simulink model "plan_nika"  (R2021b)
settings: Solver=VariableStepAuto  StartTime=0.0  StopTime=100  RelTol=1e-3
values from neighbouring files (symbols this model uses):
  cren = 0    [sis_init.m]
  g = 9.8    [sis_init.m]
  speed_tgt = 100    [sis_init.m]
  speed_tgt_2 = 130    [sis_init.m]
  v0 = 20    [sis_init.m]
undefined symbols (not defined in the file or in its folder): h0, roll
settings Model: Creator=Acer  LastModifiedBy=Acer

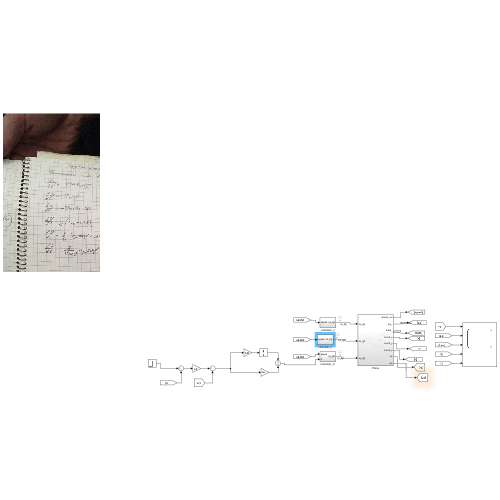
[thumbnail: Simulink's stored preview of the top-level diagram]
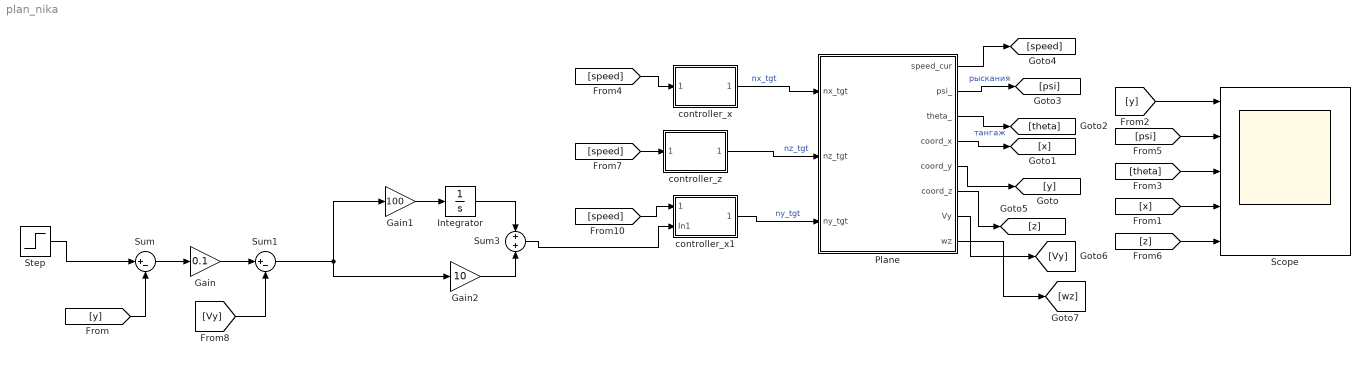
== system plan_nika ==
  Gain : Gain  Gain=0.1
  Gain1 : Gain  Gain=100
  Gain2 : Gain  Gain=10
  Integrator : Integrator
  Plane : Subsystem
  Scope : Scope  NumInputPorts=5
  Step : Step  Time=10  Before=h0  After=1500  SampleTime=0
  Sum : Sum  Inputs=|+-
  Sum1 : Sum  Inputs=|+-
  Sum3 : Sum  Inputs=+|+
  controller_x : Subsystem
  controller_x1 : Subsystem
  controller_z : Subsystem
  wires:
  controller_x/1(nx_tgt) -> Plane/1(nx_tgt)  "nx_tgt"
  Plane/5(coord_y) -> [y]
  Plane/2(psi_) -> [psi]  "рыскания"
  Plane/3(theta_) -> [theta]  "тангаж"
  Plane/4(coord_x) -> [x]
  Plane/1(speed_cur) -> [speed]
  [x] -> Scope/4
  [theta] -> Scope/3
  [speed] -> controller_x/1(speed)
  [psi] -> Scope/2
  Plane/6(coord_z) -> [z]
  [z] -> Scope/5
  [speed] -> controller_z/1(speed)
  controller_z/1(nz_tgt) -> Plane/2(nz_tgt)  "nz_tgt"
  [y] -> Scope/1
  controller_x1/1(ny_tgt) -> Plane/3(ny_tgt)  "ny_tgt"
  Step/1 -> Sum/1
  [y] -> Sum/2
  Sum/1 -> Gain/1
  Gain/1 -> Sum1/1
  Plane/7(Vy) -> [Vy]
  [Vy] -> Sum1/2
  Plane/8(wz) -> [wz]
  Integrator/1 -> Sum3/1
  Gain2/1 -> Sum3/2
  Gain1/1 -> Integrator/1
  Sum1/1 -> Gain1/1, Gain2/1
  Sum3/1 -> controller_x1/2(In1)
  [speed] -> controller_x1/1(speed)

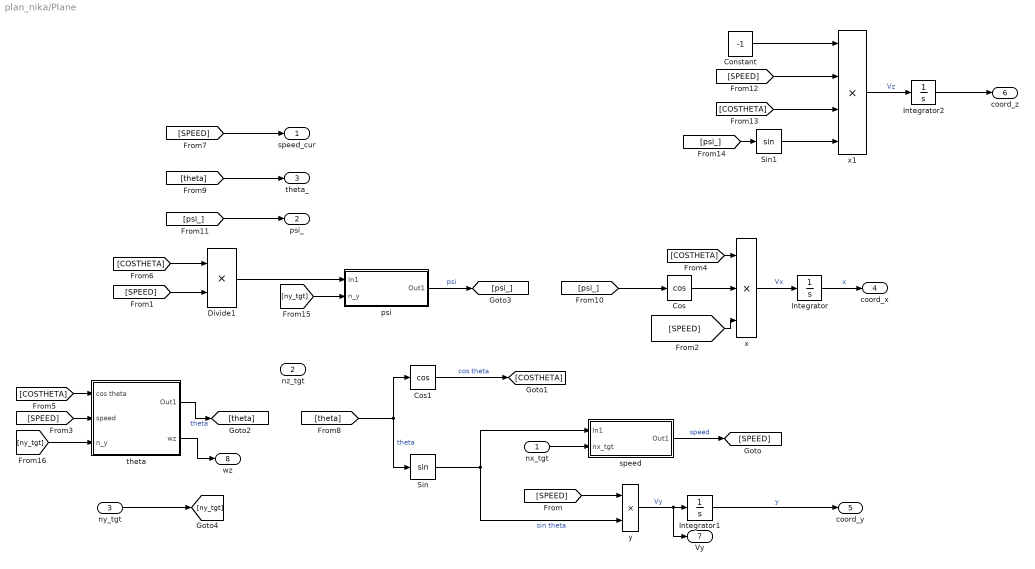
== system plan_nika/Plane ==
  nx_tgt : Inport
  nz_tgt : Inport  Port=2
  ny_tgt : Inport  Port=3
  Constant : Constant  Value=-1
  Cos : Trigonometry  Operator=cos
  Cos1 : Trigonometry  Operator=cos
  Divide1 : Product  Inputs=**
  Integrator : Integrator
  Integrator1 : Integrator  InitialCondition=h0  UpperSaturationLimit=1000
  Integrator2 : Integrator
  Sin : Trigonometry
  Sin1 : Trigonometry
  psi : Subsystem
  speed : Subsystem
  theta : Subsystem
  x : Product  Inputs=***
  x1 : Product  Inputs=****
  y : Product  Inputs=**
  speed_cur : Outport
  psi_ : Outport  Port=2
  theta_ : Outport  Port=3
  coord_x : Outport  Port=4
  coord_y : Outport  Port=5
  coord_z : Outport  Port=6
  Vy : Outport  Port=7
  wz : Outport  Port=8
  wires:
  [SPEED] -> y/1
  x/1 -> Integrator/1  "Vx"
  [COSTHETA] -> x/1
  [SPEED] -> theta/2(speed)
  [SPEED] -> Divide1/2
  y/1 -> Vy/1, Integrator1/1  "Vy"
  speed/1(Out1) -> [SPEED]  "speed"
  Sin/1 -> speed/1(In1), y/2  "sin theta"
  Divide1/1 -> psi/1(In1)
  [COSTHETA] -> Divide1/1
  [SPEED] -> x/3
  [COSTHETA] -> theta/1(cos theta)
  Cos1/1 -> [COSTHETA]  "cos theta"
  Cos/1 -> x/2
  [SPEED] -> speed_cur/1
  nx_tgt/1 -> speed/2(nx_tgt)
  Integrator/1 -> coord_x/1  "х"
  theta/1(Out1) -> [theta]  "theta"
  [theta] -> Sin/1, Cos1/1  "theta"
  [theta] -> theta_/1
  psi/1(Out1) -> [psi_]  "psi"
  [psi_] -> Cos/1
  [psi_] -> psi_/1
  [psi_] -> Sin1/1
  [SPEED] -> x1/2
  [COSTHETA] -> x1/3
  Sin1/1 -> x1/4
  Constant/1 -> x1/1
  x1/1 -> Integrator2/1  "Vz"
  Integrator2/1 -> coord_z/1
  [ny_tgt] -> psi/2(n_y)
  Integrator1/1 -> coord_y/1  "y"
  ny_tgt/1 -> [ny_tgt]
  [ny_tgt] -> theta/3(n_y)
  theta/2(wz) -> wz/1

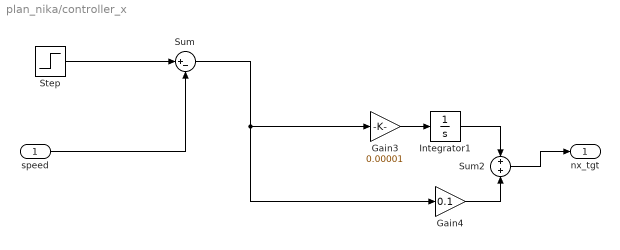
== system plan_nika/controller_x ==
  speed : Inport
  Gain3 : Gain  Gain=0.00001
  Gain4 : Gain  Gain=0.1
  Integrator1 : Integrator
  Step : Step  Time=10  Before=speed_tgt  After=speed_tgt_2  SampleTime=0
  Sum : Sum  Inputs=|+-
  Sum2 : Sum  Inputs=+|+
  nx_tgt : Outport
  wires:
  Step/1 -> Sum/1
  speed/1 -> Sum/2
  Integrator1/1 -> Sum2/1
  Gain3/1 -> Integrator1/1
  Gain4/1 -> Sum2/2
  Sum/1 -> Gain4/1, Gain3/1
  Sum2/1 -> nx_tgt/1

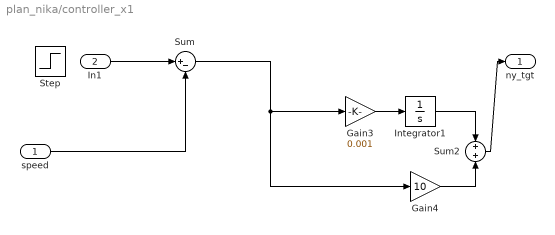
== system plan_nika/controller_x1 ==
  speed : Inport
  In1 : Inport  Port=2
  Gain3 : Gain  Gain=0.001
  Gain4 : Gain  Gain=10
  Integrator1 : Integrator
  Step : Step  Time=10  Before=speed_tgt  After=speed_tgt_2  SampleTime=0
  Sum : Sum  Inputs=|+-
  Sum2 : Sum  Inputs=+|+
  ny_tgt : Outport
  wires:
  speed/1 -> Sum/2
  In1/1 -> Sum/1
  Integrator1/1 -> Sum2/1
  Gain3/1 -> Integrator1/1
  Gain4/1 -> Sum2/2
  Sum/1 -> Gain4/1, Gain3/1
  Sum2/1 -> ny_tgt/1

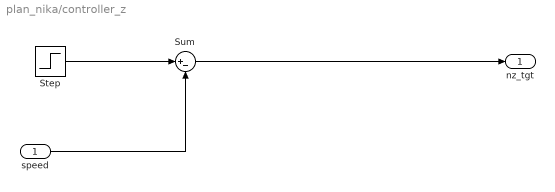
== system plan_nika/controller_z ==
  speed : Inport
  Step : Step  Time=10  Before=speed_tgt  After=speed_tgt_2  SampleTime=0
  Sum : Sum  Inputs=|+-
  nz_tgt : Outport
  wires:
  Step/1 -> Sum/1
  speed/1 -> Sum/2
  Sum/1 -> nz_tgt/1

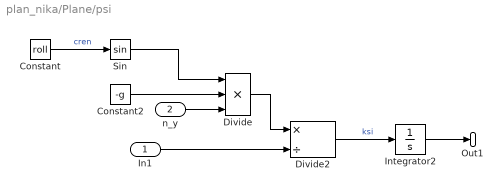
== system plan_nika/Plane/psi ==
  In1 : Inport
  n_y : Inport  Port=2
  Constant : Constant  Value=roll
  Constant2 : Constant  Value=-g
  Divide : Product  Inputs=***
  Divide2 : Product  Inputs=*/
  Integrator2 : Integrator
  Sin : Trigonometry
  Out1 : Outport
  wires:
  Divide2/1 -> Integrator2/1  "ksi"
  In1/1 -> Divide2/2
  Integrator2/1 -> Out1/1
  Constant2/1 -> Divide/2
  n_y/1 -> Divide/3
  Divide/1 -> Divide2/1
  Constant/1 -> Sin/1  "cren"
  Sin/1 -> Divide/1

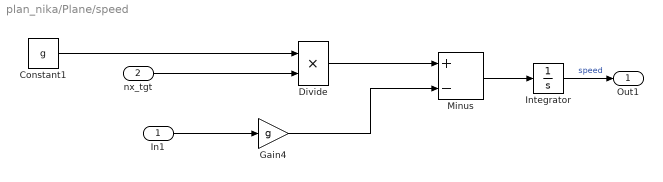
== system plan_nika/Plane/speed ==
  In1 : Inport
  nx_tgt : Inport  Port=2
  Constant1 : Constant  Value=g
  Divide : Product  Inputs=**
  Gain4 : Gain  Gain=g
  Integrator : Integrator  InitialCondition=v0
  Minus : Sum  Inputs=+-
  Out1 : Outport
  wires:
  Minus/1 -> Integrator/1
  Gain4/1 -> Minus/2
  Integrator/1 -> Out1/1  "speed"
  In1/1 -> Gain4/1
  Constant1/1 -> Divide/1
  nx_tgt/1 -> Divide/2
  Divide/1 -> Minus/1

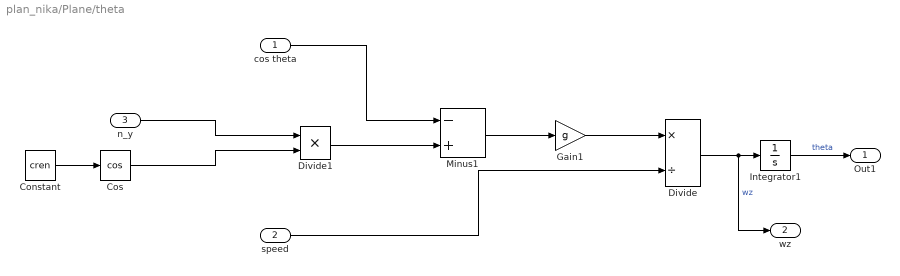
== system plan_nika/Plane/theta ==
  cos theta : Inport
  speed : Inport  Port=2
  n_y : Inport  Port=3
  Constant : Constant  Value=cren
  Cos : Trigonometry  Operator=cos
  Divide : Product  Inputs=*/
  Divide1 : Product  Inputs=**
  Gain1 : Gain  Gain=g
  Integrator1 : Integrator
  Minus1 : Sum  Inputs=-+
  Out1 : Outport
  wz : Outport  Port=2
  wires:
  Gain1/1 -> Divide/1
  Minus1/1 -> Gain1/1
  Divide/1 -> wz/1, Integrator1/1  "wz"
  Integrator1/1 -> Out1/1  "theta"
  cos theta/1 -> Minus1/1
  speed/1 -> Divide/2
  Constant/1 -> Cos/1
  n_y/1 -> Divide1/1
  Cos/1 -> Divide1/2
  Divide1/1 -> Minus1/2
